simulink library "DelayLibrary"  (R2022b)
settings: Solver=VariableStepAuto  StartTime=0.0  StopTime=10.0  RelTol=1e-3
undefined symbols (not defined in the file or in its folder): Column, delay_chain, L, max_delay, num_input_chs
libraries: FeaturePath x4, AudioStats x4, RTC x3, TuneVar x3, $bdroot x2, ITC x2, dspsigops x1, TOP x1
(part 1 of 2)
settings Model: Creator=darshana.mistry  LastModifiedBy=kl13806
settings SolverCC: AlgebraicLoopSolver=TrustRegion
settings DebuggingCC: UnconnectedInputMsg=warning  UnconnectedOutputMsg=warning  UnconnectedLineMsg=warning  SFMachineParentedDataDiag=warning  ArithmeticOperatorsInVariantConditions=warning
settings ModelReferenceCC: EnableRefExpFcnMdlSchedulingChecks=on
settings SFSimCC: CustomCodeUndefinedFunction=UseInterfaceOnly
settings RTWCC: DLArmComputeVersion=19.05

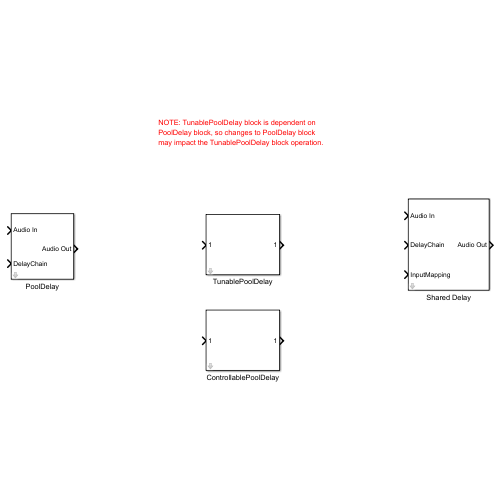
[thumbnail: Simulink's stored preview of the top-level diagram]
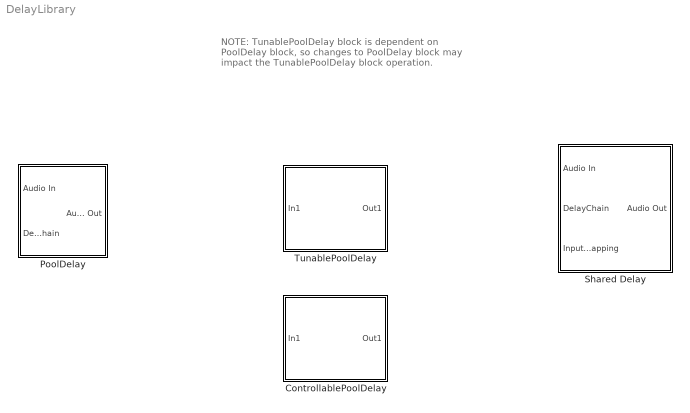
== system DelayLibrary ==
  note: NOTE: TunablePoolDelay block is dependent on
      | PoolDelay block, so changes to PoolDelay block
      | may impact the TunablePoolDelay block operation.
  ControllablePoolDelay : Subsystem  mask(Bose Tunable Pool Delay){delayType=In Samples, enableDelay=1, delaychain_var=delay_chain, maxTotalDelay=max_delay, frameSize=L, numChannels=num_input_chs, variantSelect=L2 Memory, PostOverlay=true, delayFrameLess=on, delayFrame=on, delayMultiFrame=on, FeatureName=ControllablePoolDelay, totalDelayBufferSize=0}
      mask prompts: delayType "Delay Type"; enableDelay "Enable Delay"; delaychain_var "Delay Chain for all channels (samples/ms)"; maxTotalDelay "Total Allotted Delay"; frameSize "Frame Size"; numChannels "Number Channels"; variantSelect "Implementation"; PostOverlay "Requires post-overlay action:"; delayFrameLess "delays <= frameSize"; delayFrame "frameSize < delays < (2 * frameSize)"; delayMultiFrame "delays >= (2 * frameSize)"; FeatureName "Delay name/purpose"; totalDelayBufferSize "Slow Delay Buffer Size"
      mask help:
      | 'Tunable Pool Delay' is based on 'Pool Delay' with addition of Tune and RTC parameter. Underlying block 'Pool Delay' is a multi-channel delay module with one single delay pool and adjustable delays per channel.
      | In this module, Delay chain is Tune parameter and Delay can be enabled or disabled via RTC message 'Enable_Delay'.
      mask TypeOptions delayType: In Samples | In Milliseconds
      mask TypeOptions maxTotalDelay: annDelaySubsystem/DelayEnableSubsystem/PoolDelay/maxTotalDelay | maxDelay/Value
      mask TypeOptions frameSize: annDelaySubsystem/DelayEnableSubsystem/PoolDelay/frameSize
      mask TypeOptions numChannels: annDelaySubsystem/DelayEnableSubsystem/PoolDelay/numChannels
      mask TypeOptions variantSelect: annDelaySubsystem/DelayEnableSubsystem/PoolDelay/variantSelect
      mask Callback variantSelect:
      | % Get the mask parameter value and container properties.
      | hMask = Simulink.Mask.get(gcb);
      | variant = get_param(gcb,'variantSelect');
      | container = hMask.getDialogControl('Container3');
      | 
      | % Check the value of 'variantSelect'
      | if strcmp(variant,"L2 Memory")
      |     % Set the visibility of delay panel
      |     container.Visible = 'on';
      |     MaskUtil.safe_setparam(gcbh, 'PostOverlay', 'true');
      | else
      |     % Set the visibility of delay panel
      |     container.Visible = 'off';
      |     MaskUtil.safe_setparam(gcbh, 'PostOverlay', 'false');
      | end
      mask TypeOptions PostOverlay: DelayTranslation/Delay_Samples/PostOverlay
      mask TypeOptions delayFrameLess: annDelaySubsystem/DelayEnableSubsystem/PoolDelay/delayFrameLess
      mask TypeOptions delayFrame: annDelaySubsystem/DelayEnableSubsystem/PoolDelay/delayFrame
      mask TypeOptions delayMultiFrame: annDelaySubsystem/DelayEnableSubsystem/PoolDelay/delayMultiFrame
      mask TypeOptions FeatureName: FeaturePath/FeatureName
      mask TypeOptions totalDelayBufferSize: annDelaySubsystem/DelayEnableSubsystem/PoolDelay/totalDelayBufferSize | annDelaySubsystem/DelayEnableSubsystem/PoolDelay/totalFastDelayBufferSize
      mask DialogControl Container3 Prompt: Delay Size Required
  PoolDelay : Subsystem  mask(Bose Pool Delay){variantSelect=L2 Memory, maxTotalDelay=512, delayFrameLess=on, delayFrame=on, delayMultiFrame=on, frameSize=32, numChannels=3, totalDelayBufferSize=0, totalFastDelayBufferSize=0}
      mask prompts: variantSelect "Implementation"; maxTotalDelay "Total Allotted Delay"; delayFrameLess "delays <= frameSize"; delayFrame "frameSize < delays < (2 * frameSize)"; delayMultiFrame "delays >= (2 * frameSize)"; frameSize "Frame Size"; numChannels "Number Channels"; totalDelayBufferSize "Slow Delay Buffer Size"; totalFastDelayBufferSize "Fast Delay Buffer Size"
      mask help:
      | Pool Delay is a multi-channel delay module with one single delay pool and adjustable delays per channel.  It provides support for delays greater than or equal to zero for one or more channels.  Total delay buffer size is the sum of all channel delays.  The Pool Delay model supports three different implementations, selectable from the model mask:
      |
      | - L1 Memory:  Optimized CRL (Code Replacement Library) code running on core with delay buffer in L1 Memory
      | - L2 Memory:  Optimized CRL code running on core and using DMA for memory copies with primary delay buffer in L2 Memory
      | - Generic:  Generic Matlab implementation running on core for targets without CRL support
      |
      | This model has two inputs and one output:
      |
      | - AudioIn [in]:  Audio input stream containing audio frame samples for one or more channels  [frameSize x numChannels]
      | - Delay [in]:  Delay in samples for each channel  [1 x numChannels]
      | - AudioOut [out]:  Audio output stream containing delayed audio frame samples for one or more channels  [frameSize x numChannels]
      |
      | NOTE: The Pool Delay codeWorkMemory buffer should always be mapped to L1 memory or core MIPS usage will increase.
      |
      | For more information, please see 'Help'.
      mask init:
      | % Create alias for delay buffer for each instance of model
      | PoolDelayMask(gcbh, variantSelect);
      | 
      | % There are three implementation types:
      | % Type    Value  Description
      | % L1 Memory  1      Optimized CRL code running on core with delay buffer
      | %                   in L1 Memory
      | % L2 Memory  2      Optimized CRL code running on core and using DMA for 
      | %                   memory copies with primary delay buffer in L2 Memory
      | % GENERIC    3      Generic Matlab implementation running on core for 
      | %                   other targets without CRL support
      | 
      | if variantSelect == 1
      |     % L1 Memory Core Implementation
      |     
      |     % Set delay buffer sizes. Only fast delay buffer (L1) is used for  
      |     % core implementation.
      |     totalFastDelayBufferSize = maxTotalDelay;
      |     totalDelayBufferSize =  2;      % Eliminates scaler CRL table entry
      |     
      |     % CRL code work memory size in bytes is equal to:
      |     %             sizeof(coreWorkMemory_t);
      |     % No variable data memory is used.  NOTE: This must be updated to 
      |     % match the CRL code if any changes are made to the coreWorkMemory_t 
      |     % structure.
      |     codeWorkMemorySize = (36/4);  % Size in words
      |     
      | elseif variantSelect == 2
      |     % L2 Memory DMA Implementation
      | 
      |     % Set delay buffer sizes. Total delay memory is split between
      |     % the delay buffer and fast delay buffer, with only 1 frame of
      |     % samples, or the delay (delay < frameSize) for each channel 
      |     % stored in the fast delay buffer. Get the delay buffer sizes and
      |     % DMA TCB memory required for the worst case Room Mode Down Load
      |     % given the specified delay categories and maxTotalDelay.
      |     delayConfig = [delayFrameLess, delayFrame, delayMultiFrame];
      |     [totalFastDelayBufferSize, totalDelayBufferSize, ...
      |      maxTcbMemSize, maxChanMapSize] = ...
      |             PoolDelayDmaMemorySizes(delayConfig, maxTotalDelay, ...
      |                                     numChannels, frameSize);
      |     
      |     % Make sure circular delay buffer size is at least as large as the
      |     % frame size. Note this is required to ensure the SHARC built-in
      |     % circindex() function works correctly in the CRL code.
      |     totalDelayBufferSize = max(frameSize, totalDelayBufferSize);
      |     
      |     % CRL code work memory size in bytes is equal to:
      |     %             sizeof(dmaWorkMemory_t) + variableDataSize;
      |     % with variable data size dependent on number channels and number
      |     % DMA TCB blocks.  NOTE: This must be updated to match the CRL code
      |     % if any changes are made to the dmaWorkMemory_t structure.
      |     codeWorkMemorySize = (156/4) + maxTcbMemSize + maxChanMapSize; % Size in words
      |     
      | else
      |     % Generic Implementation
      |     
      |     % Set delay buffer sizes. Only fast delay buffer (L1) is used for
      |     % generic implementation.
      |     totalFastDelayBufferSize = maxTotalDelay;
      |     totalDelayBufferSize =  1;    
      |     
      |     % This is not used if there is no CRL
      |     codeWorkMemorySize = 1;
      | end
      mask Help:
      | Help on Mask Parameters:
      | 
      | All variants of the model contain the following mask parameters:
      | 
      | - Implementation:  Selects the desired model implementation to use (L1 Memory, L2 Memory, or Generic)
      | - Total Allotted Delay:  The provides delay buffer sizing for the maximum Room Model Down Load (RMDL) or non-RMDL delay configuration required.  It is the sum of all channels delays in samples for the largest RMDL delay case.  (scalar)
      | - Frame Size:  Specifies the audio frame size in samples (scalar)
      | - Number Channels:  Specifies the number of channel and applies to the audio input, output, and delay channels (scalar)
      | 
      | The 'L2 Memory' implementation contains the following additional mask parameter:
      | 
      | - Delay Sizes Required: The appropriate check boxes must be checked to specify delay categories required.  Delay categories include the following: (delays <= frameSize), (frameSize < delays < (2 * frameSize)), and (delays >= (2 * frameSize).  The correct selection of these delay categories is required to ensure the delay buffers and other model data is sized correctly.
      | 
      | Note that since the 'L2 Memory' implementations takes advantage of DMA memory copies performed by the hardware DMA engine, the implementation differs from the other model implementations and in order to minimize the memory usage required to support all channel delay configurations, the channel delay categories required must be known.  The specific delay cases required for RMDL and non-RMDL model instances determine overall memory required for delay buffers and DMA descriptor memory.
      | 
      | Mask Usage Example:
      | 
      | 3 input and output channels, with channel delays of 16, 48, 80 samples for a case that does not require RMDL, and a frame size of 32 samples.
      | 
      | For example, to use the  L1 Memory implementation, set the mask parameters as follows:
      | 
      | Implementation = 'L1 Memory'
      | Total RMDL Allotted Delay = 148        (16 + 48 + 80)
      | Frame Size = 32
      | Number Channels = 3
      | 
      | For the same example with the L2 Memory implementation, set all the above parameters as stated, except with:
      | 
      | Implementation = 'L2 Memory'
      | Delay Sizes Required should have all delay categories checked, as the delays of 16, 48, 80 include all categories.  These parameters and the Total Allotted Delay are used size memory to support the delay configuration.  If for example, all delays required were less than equal to a frame only that delay category should be checked.
      | 
      | Note that 'Delay Sizes Required' is specific to the L2 Memory implementation and does not apply to the other implementations.
      | 
      | The 'Generic' implementation would require the identical mask parameter initialization as the L1 memory implementation, except with:
      | 
      | Implementation = 'Generic'
      mask TypeOptions variantSelect: L1 Memory | L2 Memory | Generic
      mask Callback variantSelect:
      | % Get the mask parameter value and container properties.
      | hMask = Simulink.Mask.get(gcb);
      | variant = get_param(gcb,'variantSelect');
      | container = hMask.getDialogControl('DelayPanel');
      | 
      | % Check the value of 'variantSelect'
      | if strcmp(variant,"L2 Memory")
      |     % Set the visibility of delay panel
      |     container.Visible = 'on';
      | else
      |     % Set the visibility of delay panel
      |     container.Visible = 'off';
      | end
      mask DialogControl DelayPanel Prompt: Delay Sizes Required
  Shared Delay : Subsystem  mask(Bose Shared Delay){maxTotalDelay=512, frameSize=32, numInputs=2, numOutputs=3, totalDelayBufferSize=0, fastDmaBufferSize=0}
      mask prompts: maxTotalDelay "Total Allotted Delay"; frameSize "Frame Size"; numInputs "Number Inputs"; numOutputs "Number Outputs"; totalDelayBufferSize "Slow Delay Buffer Size"; fastDmaBufferSize "Fast DMA Buffer Size"
      mask help:
      | Shared Delay is a multi-input channel delay module with one or more adjustable output delay taps per input channel, based on how input channels are mapped to outputs.  It provides support for delays greater than or equal to zero.  The Shared Delay model supports only one implementation.  It is a DMA based write before delay buffer read implementation, with total delay buffer size of the sum of the maximum output channel tap delay for each input channel, plus one frame size per input channel.
      |
      | This model has two inputs and one output:
      |
      | - AudioIn [in]:  Audio input stream containing audio frame samples for one or more input channels  [frameSize x numInputs]
      | - DelayChain [in]:  Delay in samples for all input channel's output tap channels  [1 x numOutputs]
      | - InputMapping [in]:  Zero based mapping of input channels to output tap channels  [1 x numOutputs]
      | - AudioOut [out]:  Audio output stream containing delayed audio frame samples for one or more output channels  [frameSize x numOutputs]
      |
      | The delay buffer can be mapped to L3, L2 or L1 memory with proper definition of the code generated pragma section memory mappings.
      |
      | NOTE: The Shared Delay codeWorkMemory buffer should always be mapped to L1 memory or core MIPS usage will increase.
      |
      | For more information, please see 'Help'.
      mask init:
      | % Create alias for delay buffer for each instance of model
      | SharedDelayMask(gcbh);
      | 
      | % Set delay buffer size and fast DMA output buffer size. These
      | % are worst case Room Mode Down Load sizes given maxTotalDelay.
      | totalDelayBufferSize = maxTotalDelay + (numInputs * frameSize);
      | fastDmaBufferSize = numOutputs * frameSize;
      | 
      | % CRL code work memory size in bytes is equal to:
      | %             sizeof(dmaWorkMemory_t) + variableDataSize;
      | % with variable data size dependent on number channels and number
      | % DMA TCB blocks.  NOTE: This must be updated to match the CRL code
      | % if any changes are made to the dmaWorkMemory_t structure.
      | codeWorkMemorySize = (160/4) + (numInputs * (14 + 5)) + ...
      |                      (2 * numOutputs);    % Size in words
      mask Help:
      | Help on Mask Parameters:
      | 
      | The Shared Delay model contains the following mask parameters:
      | 
      | - Total Allotted Delay:  Specifies delay buffer sizing for the maximum Room Model Down Load (RMDL) or non-RMDL delay configuration required.  It is the sum of the maximum output channel tap delay for each input channel in samples that supports the largest RMDL delay case.  (scalar)
      | - Frame Size:  Specifies the audio frame size in samples (scalar)
      | - Number Input Channels:  Specifies the number of input channels and applies to the audio inputs (scalar)
      | - Number Output Channels:  Specifies the number of output channels and applies to the audio outputs, delays and input mapping (scalar)
      | 
      | Mask Usage Example:
      | 
      | 2 input channels, with output channel tap delays of 16, 48, 80 samples for input 1 and output channel tap delays of 37, 62 samples for input channel 2.    Assumption is this case does not require RMDL and the frame size is 32 samples.
      | 
      | For this example, set the mask parameters and inputs as follows:
      | 
      | Total Allotted Delay = 142        max( [16 48 80] ) + max( [37  62] ) = 80 + 62
      | Frame Size = 32
      | Number Inputs = 2
      | Number Outputs = 5                (3 + 2)
      | 
      | DelayChain = [16 48 80 37 62]
      | InputMapping = [0 0 0 1 1]
  TunablePoolDelay : Subsystem  mask(Bose Tunable Pool Delay){delayType=In Samples, enableDelay=1, delaychain_var=delay_chain, maxTotalDelay=max_delay, frameSize=L, numChannels=num_input_chs, variantSelect=L2 Memory, PostOverlay=true, delayFrameLess=on, delayFrame=on, delayMultiFrame=on, FeatureName=TunablePoolDelay, totalDelayBufferSize=0}
      mask prompts: delayType "Delay Type"; enableDelay "Enable Delay"; delaychain_var "Delay Chain for all channels (samples/ms)"; maxTotalDelay "Total Allotted Delay"; frameSize "Frame Size"; numChannels "Number Channels"; variantSelect "Implementation"; PostOverlay "Requires post-overlay action:"; delayFrameLess "delays <= frameSize"; delayFrame "frameSize < delays < (2 * frameSize)"; delayMultiFrame "delays >= (2 * frameSize)"; FeatureName "Delay name/purpose"; totalDelayBufferSize "Slow Delay Buffer Size"
      mask help:
      | 'Tunable Pool Delay' is based on 'Pool Delay' with addition of Tune and RTC parameter. Underlying block 'Pool Delay' is a multi-channel delay module with one single delay pool and adjustable delays per channel.
      | In this module, Delay chain is Tune parameter and Delay can be enabled or disabled via RTC message 'Enable_Delay'.
      mask TypeOptions delayType: In Samples | In Milliseconds
      mask TypeOptions maxTotalDelay: annDelaySubsystem/DelayEnableSubsystem/PoolDelay/maxTotalDelay | maxDelay/Value
      mask TypeOptions frameSize: annDelaySubsystem/DelayEnableSubsystem/PoolDelay/frameSize
      mask TypeOptions numChannels: annDelaySubsystem/DelayEnableSubsystem/PoolDelay/numChannels
      mask TypeOptions variantSelect: annDelaySubsystem/DelayEnableSubsystem/PoolDelay/variantSelect
      mask Callback variantSelect:
      | % Get the mask parameter value and container properties.
      | hMask = Simulink.Mask.get(gcb);
      | variant = get_param(gcb,'variantSelect');
      | container = hMask.getDialogControl('Container3');
      | 
      | % Check the value of 'variantSelect'
      | if strcmp(variant,"L2 Memory")
      |     % Set the visibility of delay panel
      |     container.Visible = 'on';
      |     MaskUtil.safe_setparam(gcbh, 'PostOverlay', 'true');
      | else
      |     % Set the visibility of delay panel
      |     container.Visible = 'off';
      |     MaskUtil.safe_setparam(gcbh, 'PostOverlay', 'false');
      | end
      mask TypeOptions PostOverlay: DelayTranslation/Delay_Samples/PostOverlay
      mask TypeOptions delayFrameLess: annDelaySubsystem/DelayEnableSubsystem/PoolDelay/delayFrameLess
      mask TypeOptions delayFrame: annDelaySubsystem/DelayEnableSubsystem/PoolDelay/delayFrame
      mask TypeOptions delayMultiFrame: annDelaySubsystem/DelayEnableSubsystem/PoolDelay/delayMultiFrame
      mask TypeOptions FeatureName: FeaturePath/FeatureName
      mask TypeOptions totalDelayBufferSize: annDelaySubsystem/DelayEnableSubsystem/PoolDelay/totalDelayBufferSize | annDelaySubsystem/DelayEnableSubsystem/PoolDelay/totalFastDelayBufferSize
      mask DialogControl Container3 Prompt: Delay Size Required

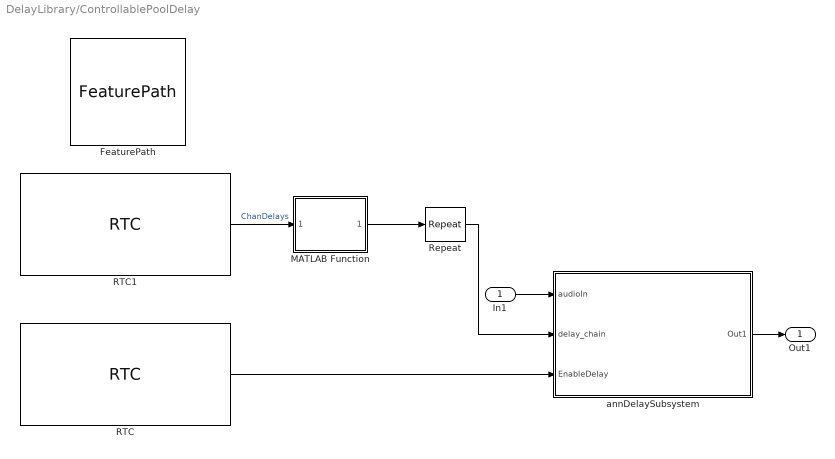
== system DelayLibrary/ControllablePoolDelay ==
  In1 : Inport
  FeaturePath : FeaturePath/FeaturePath  FeatureName=ControllablePoolDelay  IsGroup=off  GroupNumber=-1  IsModule=off  TriggerInit=[-120 -76 -5 31]
      settings: SourceProductName=Bose Talaria
  MATLAB Function : MATLAB Function  TreatAsAtomicUnit=on
  RTC : RTC/RTC  REQ_Priority=RTC_Mask.NormalPriority  RequestAtInit=off  EnableRequest=off  REQElemName1=Enable_annDelay  REQElemType1=uint32  REQElemWidth1=1  REQElemInitial1=enableDelay  REQElemType2=uint32  REQElemWidth2=1  REQElemInitial2=[]  REQElemType3=uint32  REQElemWidth3=1  REQElemInitial3=[]  REQElemType4=uint32  REQElemWidth4=1  REQElemInitial4=[]  REQElemType5=uint32  REQElemWidth5=1  REQElemInitial5=[]  REQElemType6=uint32  REQElemWidth6=1  REQElemInitial6=[]  REQElemType7=uint32  REQElemWidth7=1  REQElemInitial7=[]  REQElemType8=uint32  REQElemWidth8=1  REQElemInitial8=[]  REQElemType9=uint32  REQElemWidth9=1  REQElemInitial9=[]  REQElemType10=uint32  REQElemWidth10=1  REQElemInitial10=[]  EnableResponse=on  EnableRSP_StatusIn=off  RSPElemType1=uint32  RSPElemWidth1=1  RSPElemType2=uint32  RSPElemWidth2=1  RSPElemType3=uint32  RSPElemWidth3=1  RSPElemType4=uint32  RSPElemWidth4=1  RSPElemType5=uint32  RSPElemWidth5=1  RSPElemType6=uint32  RSPElemWidth6=1  RSPElemType7=uint32  RSPElemWidth7=1  RSPElemType8=uint32  RSPElemWidth8=1  RSPElemType9=uint32  RSPElemWidth9=1  RSPElemType10=uint32  RSPElemWidth10=1  EnableNotification=off  EnableNTF_PrepTrig=off  NTFElemType1=uint32  NTFElemWidth1=1  NTFElemType2=uint32  NTFElemWidth2=1  NTFElemType3=uint32  NTFElemWidth3=1  NTFElemType4=uint32  NTFElemWidth4=1  NTFElemType5=uint32  NTFElemWidth5=1  NTFElemType6=uint32  NTFElemWidth6=1  NTFElemType7=uint32  NTFElemWidth7=1  NTFElemType8=uint32  NTFElemWidth8=1  NTFElemType9=uint32  NTFElemWidth9=1  NTFElemType10=uint32  NTFElemWidth10=1  MaskMessageName=Enable_Delay
      settings: SourceProductName=Bose Talaria
  RTC1 : RTC/RTC  REQ_Priority=RTC_Mask.NormalPriority  RequestAtInit=off  EnableRequest=off  REQElemName1=Delay_value  REQElemType1=uint32  REQElemWidth1=1  REQElemInitial1=delaychain_var  REQElemType2=uint32  REQElemWidth2=1  REQElemInitial2=[]  REQElemType3=uint32  REQElemWidth3=1  REQElemInitial3=[]  REQElemType4=uint32  REQElemWidth4=1  REQElemInitial4=[]  REQElemType5=uint32  REQElemWidth5=1  REQElemInitial5=[]  REQElemType6=uint32  REQElemWidth6=1  REQElemInitial6=[]  REQElemType7=uint32  REQElemWidth7=1  REQElemInitial7=[]  REQElemType8=uint32  REQElemWidth8=1  REQElemInitial8=[]  REQElemType9=uint32  REQElemWidth9=1  REQElemInitial9=[]  REQElemType10=uint32  REQElemWidth10=1  REQElemInitial10=[]  EnableResponse=on  EnableRSP_StatusIn=off  RSPElemType1=uint32  RSPElemWidth1=1  RSPElemType2=uint32  RSPElemWidth2=1  RSPElemType3=uint32  RSPElemWidth3=1  RSPElemType4=uint32  RSPElemWidth4=1  RSPElemType5=uint32  RSPElemWidth5=1  RSPElemType6=uint32  RSPElemWidth6=1  RSPElemType7=uint32  RSPElemWidth7=1  RSPElemType8=uint32  RSPElemWidth8=1  RSPElemType9=uint32  RSPElemWidth9=1  RSPElemType10=uint32  RSPElemWidth10=1  EnableNotification=off  EnableNTF_PrepTrig=off  NTFElemType1=uint32  NTFElemWidth1=1  NTFElemType2=uint32  NTFElemWidth2=1  NTFElemType3=uint32  NTFElemWidth3=1  NTFElemType4=uint32  NTFElemWidth4=1  NTFElemType5=uint32  NTFElemWidth5=1  NTFElemType6=uint32  NTFElemWidth6=1  NTFElemType7=uint32  NTFElemWidth7=1  NTFElemType8=uint32  NTFElemWidth8=1  NTFElemType9=uint32  NTFElemWidth9=1  NTFElemType10=uint32  NTFElemWidth10=1  MaskMessageName=Delay_value
      settings: SourceProductName=Bose Talaria
  Repeat : dspsigops/Repeat  N=numChannels  InputProcessing=Columns as channels (frame based)  RateOptions=Enforce single-rate processing  ic=0  mode=Unused parameter value
  annDelaySubsystem : Subsystem
  Out1 : Outport  VectorParamsAs1DForOutWhenUnconnected=off
  wires:
  In1/1 -> annDelaySubsystem/1(audioIn)
  annDelaySubsystem/1(Out1) -> Out1/1
  RTC1/1 -> MATLAB Function/1(Amount)  "ChanDelays"
  Repeat/1 -> annDelaySubsystem/2(delay_chain)
  RTC/1 -> annDelaySubsystem/3(EnableDelay)
  MATLAB Function/1(Samples) -> Repeat/1

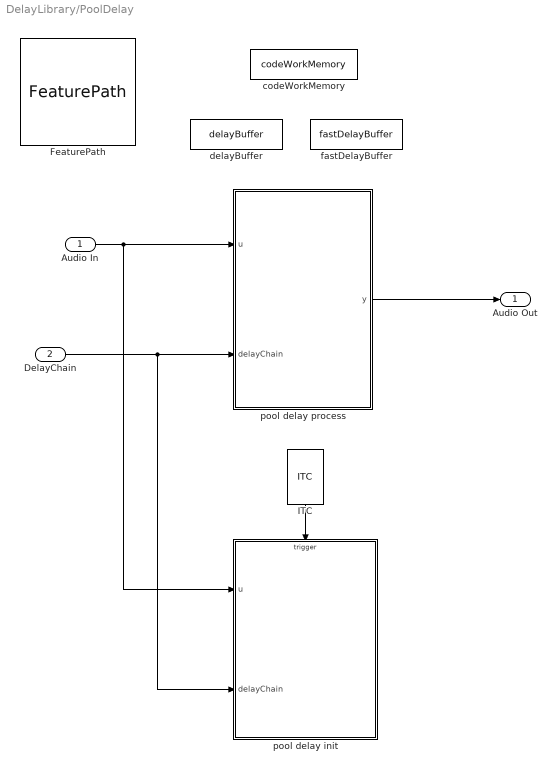
== system DelayLibrary/PoolDelay ==
  Audio In : Inport
  DelayChain : Inport  Port=2  OutDataTypeStr=uint32  PortDimensions=[1, numChannels]
  FeaturePath : FeaturePath/FeaturePath  FeatureName=PoolDelay  IsGroup=off  GroupNumber=-1  IsModule=off  TriggerInit=[205 -116 320 -9]
      settings: SourceProductName=Bose Talaria
  ITC : ITC/ITC
      settings: SourceProductName=Bose Talaria
  codeWorkMemory : DataStoreMemory  DataStoreName=codeWorkMemory  WriteAfterWriteMsg=warning  InitialValue=zeros(1,codeWorkMemorySize)  EmbeddedSignalClassName=Blocklib.Signal  ShowAdditionalParam=off  OutDataTypeStr=uint32
  delayBuffer : DataStoreMemory  DataStoreName=delayBuffer  ReadBeforeWriteMsg=warning  WriteAfterWriteMsg=warning  WriteAfterReadMsg=warning  InitialValue=zeros(totalDelayBufferSize,1)  EmbeddedSignalClassName=Blocklib.Signal  ShowAdditionalParam=off  OutDataTypeStr=single
  fastDelayBuffer : DataStoreMemory  DataStoreName=fastDelayBuffer  ReadBeforeWriteMsg=warning  WriteAfterWriteMsg=warning  WriteAfterReadMsg=warning  InitialValue=zeros(totalFastDelayBufferSize,1)  EmbeddedSignalClassName=Blocklib.Signal  ShowAdditionalParam=off  OutDataTypeStr=single
  pool delay init : MATLAB Function  TreatAsAtomicUnit=on  RTWFcnName=foo
  pool delay process : MATLAB Function  TreatAsAtomicUnit=on
  Audio Out : Outport  VectorParamsAs1DForOutWhenUnconnected=off
  wires:
  ITC/1 -> pool delay init/Trigger
  pool delay process/1(y) -> Audio Out/1
  Audio In/1 -> pool delay process/1(u), pool delay init/1(u)
  DelayChain/1 -> pool delay init/2(delayChain), pool delay process/2(delayChain)

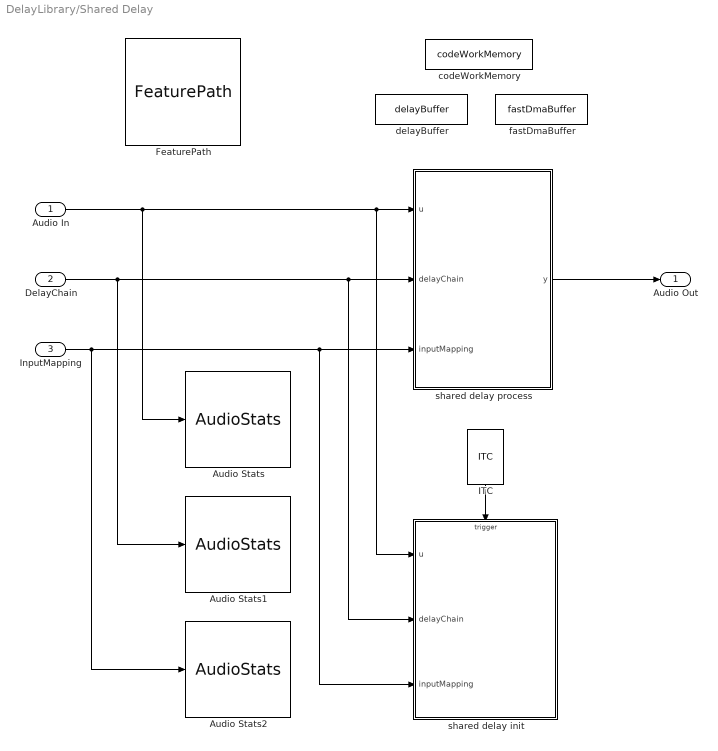
== system DelayLibrary/Shared Delay ==
  Audio In : Inport
  DelayChain : Inport  Port=2  OutDataTypeStr=int32  PortDimensions=[1, numOutputs]
  InputMapping : Inport  Port=3  OutDataTypeStr=int32  PortDimensions=[1 numOutputs]
  Audio Stats : AudioStats/AudioStats  DoSampleRate=off  TypeSampleRate=Inherit: auto  DoCallRate=off  TypeCallRate=Inherit: auto  DoFrameSize=off  TypeFrameSize=Inherit: auto  DoChannelCount=off  TypeChannelCount=Inherit: auto  DoTaskRateFactor=off  TypeTaskRateFactor=Inherit: auto  MacroNameRoot=AUDIO  MacroNameRootEval='AUDIO'  IsMacroNameEval=off  MacroSampleRate=off  MacroCallRate=off  MacroFrameSize=off  MacroChannelCount=off  MacroTaskRateFactor=off  MacroTaskId=off  ValidateSampleRate=off  ValueSampleRate=[]  ValidateCallRate=off  ValueCallRate=[]  ValidateFrameSize=on  ValueFrameSize=frameSize  ValidateChannelCount=on  ValueChannelCount=numInputs  ValidateTaskRateFactor=off  ValueTaskRateFactor=[]
      settings: SourceProductName=Bose Talaria
  Audio Stats1 : AudioStats/AudioStats  DoSampleRate=off  TypeSampleRate=Inherit: auto  DoCallRate=off  TypeCallRate=Inherit: auto  DoFrameSize=off  TypeFrameSize=Inherit: auto  DoChannelCount=off  TypeChannelCount=Inherit: auto  DoTaskRateFactor=off  TypeTaskRateFactor=Inherit: auto  MacroNameRoot=AUDIO  MacroNameRootEval='AUDIO'  IsMacroNameEval=off  MacroSampleRate=off  MacroCallRate=off  MacroFrameSize=off  MacroChannelCount=off  MacroTaskRateFactor=off  MacroTaskId=off  ValidateSampleRate=off  ValueSampleRate=[]  ValidateCallRate=off  ValueCallRate=[]  ValidateFrameSize=off  ValueFrameSize=[]  ValidateChannelCount=on  ValueChannelCount=numOutputs  ValidateTaskRateFactor=off  ValueTaskRateFactor=[]
      settings: SourceProductName=Bose Talaria
  Audio Stats2 : AudioStats/AudioStats  DoSampleRate=off  TypeSampleRate=Inherit: auto  DoCallRate=off  TypeCallRate=Inherit: auto  DoFrameSize=off  TypeFrameSize=Inherit: auto  DoChannelCount=off  TypeChannelCount=Inherit: auto  DoTaskRateFactor=off  TypeTaskRateFactor=Inherit: auto  MacroNameRoot=AUDIO  MacroNameRootEval='AUDIO'  IsMacroNameEval=off  MacroSampleRate=off  MacroCallRate=off  MacroFrameSize=off  MacroChannelCount=off  MacroTaskRateFactor=off  MacroTaskId=off  ValidateSampleRate=off  ValueSampleRate=[]  ValidateCallRate=off  ValueCallRate=[]  ValidateFrameSize=off  ValueFrameSize=[]  ValidateChannelCount=on  ValueChannelCount=numOutputs  ValidateTaskRateFactor=off  ValueTaskRateFactor=[]
      settings: SourceProductName=Bose Talaria
  FeaturePath : FeaturePath/FeaturePath  FeatureName=SharedDelay  IsGroup=off  GroupNumber=-1  IsModule=off  TriggerInit=[310 -96 425 11]
      settings: SourceProductName=Bose Talaria
  ITC : ITC/ITC
      settings: SourceProductName=Bose Talaria
  codeWorkMemory : DataStoreMemory  DataStoreName=codeWorkMemory  WriteAfterWriteMsg=warning  InitialValue=zeros(1,codeWorkMemorySize)  EmbeddedSignalClassName=Blocklib.Signal  ShowAdditionalParam=off  OutDataTypeStr=uint32
  delayBuffer : DataStoreMemory  DataStoreName=delayBuffer  ReadBeforeWriteMsg=warning  WriteAfterWriteMsg=warning  WriteAfterReadMsg=warning  InitialValue=zeros(totalDelayBufferSize,1)  EmbeddedSignalClassName=Blocklib.Signal  ShowAdditionalParam=off  OutDataTypeStr=single
  fastDmaBuffer : DataStoreMemory  DataStoreName=fastDmaBuffer  ReadBeforeWriteMsg=warning  WriteAfterWriteMsg=warning  WriteAfterReadMsg=warning  InitialValue=zeros(fastDmaBufferSize,1)  EmbeddedSignalClassName=Blocklib.Signal  ShowAdditionalParam=off  OutDataTypeStr=single
  shared delay init : MATLAB Function  TreatAsAtomicUnit=on  RTWFcnName=foo
  shared delay process : MATLAB Function  TreatAsAtomicUnit=on
  Audio Out : Outport  VectorParamsAs1DForOutWhenUnconnected=off
  wires:
  Audio In/1 -> shared delay process/1(u), shared delay init/1(u), Audio Stats/1
  InputMapping/1 -> shared delay process/3(inputMapping), shared delay init/3(inputMapping), Audio Stats2/1
  ITC/1 -> shared delay init/Trigger
  shared delay process/1(y) -> Audio Out/1
  DelayChain/1 -> shared delay process/2(delayChain), shared delay init/2(delayChain), Audio Stats1/1

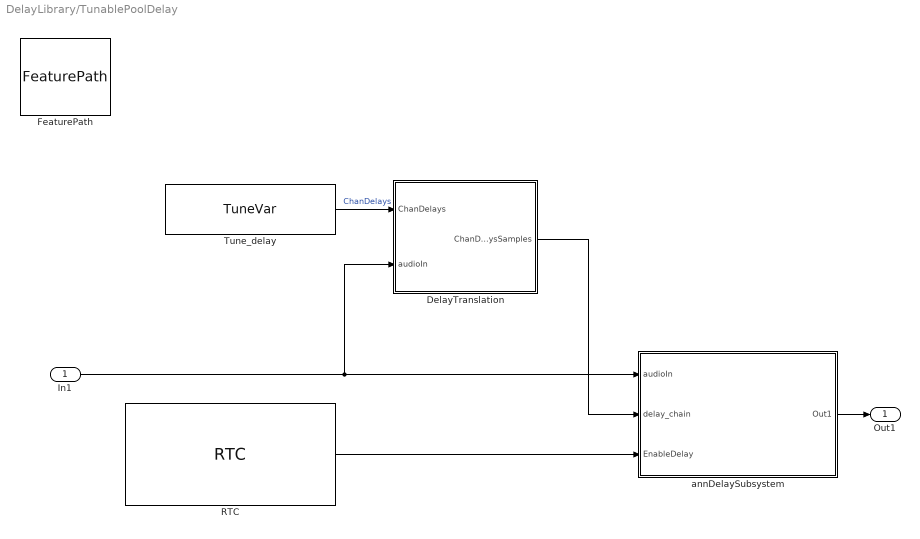
== system DelayLibrary/TunablePoolDelay ==
  In1 : Inport
  DelayTranslation : Subsystem
  FeaturePath : FeaturePath/FeaturePath  FeatureName=TunablePoolDelay  IsGroup=off  GroupNumber=-1  IsModule=off  TriggerInit=[-255 -156 -165 -79]
      settings: SourceProductName=Bose Talaria
  RTC : RTC/RTC  REQ_Priority=RTC_Mask.NormalPriority  RequestAtInit=off  EnableRequest=off  REQElemName1=Enable_annDelay  REQElemType1=uint32  REQElemWidth1=1  REQElemInitial1=enableDelay  REQElemType2=uint32  REQElemWidth2=1  REQElemInitial2=[]  REQElemType3=uint32  REQElemWidth3=1  REQElemInitial3=[]  REQElemType4=uint32  REQElemWidth4=1  REQElemInitial4=[]  REQElemType5=uint32  REQElemWidth5=1  REQElemInitial5=[]  REQElemType6=uint32  REQElemWidth6=1  REQElemInitial6=[]  REQElemType7=uint32  REQElemWidth7=1  REQElemInitial7=[]  REQElemType8=uint32  REQElemWidth8=1  REQElemInitial8=[]  REQElemType9=uint32  REQElemWidth9=1  REQElemInitial9=[]  REQElemType10=uint32  REQElemWidth10=1  REQElemInitial10=[]  EnableResponse=on  EnableRSP_StatusIn=off  RSPElemType1=uint32  RSPElemWidth1=1  RSPElemType2=uint32  RSPElemWidth2=1  RSPElemType3=uint32  RSPElemWidth3=1  RSPElemType4=uint32  RSPElemWidth4=1  RSPElemType5=uint32  RSPElemWidth5=1  RSPElemType6=uint32  RSPElemWidth6=1  RSPElemType7=uint32  RSPElemWidth7=1  RSPElemType8=uint32  RSPElemWidth8=1  RSPElemType9=uint32  RSPElemWidth9=1  RSPElemType10=uint32  RSPElemWidth10=1  EnableNotification=off  EnableNTF_PrepTrig=off  NTFElemType1=uint32  NTFElemWidth1=1  NTFElemType2=uint32  NTFElemWidth2=1  NTFElemType3=uint32  NTFElemWidth3=1  NTFElemType4=uint32  NTFElemWidth4=1  NTFElemType5=uint32  NTFElemWidth5=1  NTFElemType6=uint32  NTFElemWidth6=1  NTFElemType7=uint32  NTFElemWidth7=1  NTFElemType8=uint32  NTFElemWidth8=1  NTFElemType9=uint32  NTFElemWidth9=1  NTFElemType10=uint32  NTFElemWidth10=1  MaskMessageName=Enable_Delay
      settings: SourceProductName=Bose Talaria
  Tune_delay : TuneVar/TuneVar  TuneName=ChanDelays  SpecifyMaxSize=off  VariableDim=2 (Column)  MaxSize=[1 1]  TunabilityNumber=1  MinValue=[]  MaxValue=[]  TriggerInit=[-110 -10 60 40]  MaskValue=delaychain_var
      settings: SourceProductName=Bose Talaria
  annDelaySubsystem : Subsystem
  Out1 : Outport  VectorParamsAs1DForOutWhenUnconnected=off
  wires:
  RTC/1 -> annDelaySubsystem/3(EnableDelay)
  DelayTranslation/1(ChanDelaysSamples) -> annDelaySubsystem/2(delay_chain)
  Tune_delay/1 -> DelayTranslation/1(ChanDelays)  "ChanDelays"
  annDelaySubsystem/1(Out1) -> Out1/1
  In1/1 -> annDelaySubsystem/1(audioIn), DelayTranslation/2(audioIn)

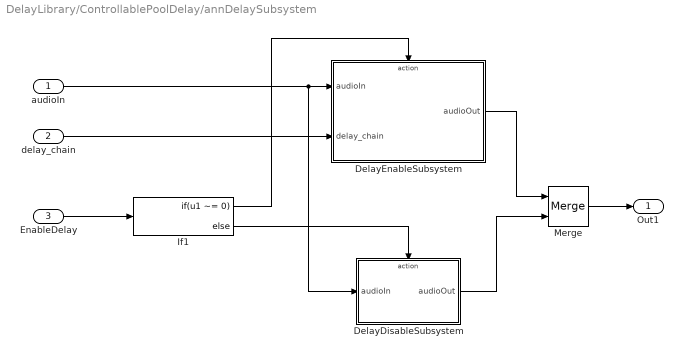
== system DelayLibrary/ControllablePoolDelay/annDelaySubsystem ==
  audioIn : Inport
  delay_chain : Inport  Port=2
  EnableDelay : Inport  Port=3
  DelayDisableSubsystem : Subsystem  TreatAsAtomicUnit=on
  DelayEnableSubsystem : Subsystem  TreatAsAtomicUnit=on
  If1 : If  IfExpression=u1 ~= 0
  Merge : Merge
  Out1 : Outport  VectorParamsAs1DForOutWhenUnconnected=off
  wires:
  EnableDelay/1 -> If1/1
  If1/1 -> DelayEnableSubsystem/Action
  audioIn/1 -> DelayDisableSubsystem/1(audioIn), DelayEnableSubsystem/1(audioIn)
  delay_chain/1 -> DelayEnableSubsystem/2(delay_chain)
  DelayEnableSubsystem/1(audioOut) -> Merge/1
  If1/2 -> DelayDisableSubsystem/Action
  Merge/1 -> Out1/1
  DelayDisableSubsystem/1(audioOut) -> Merge/2

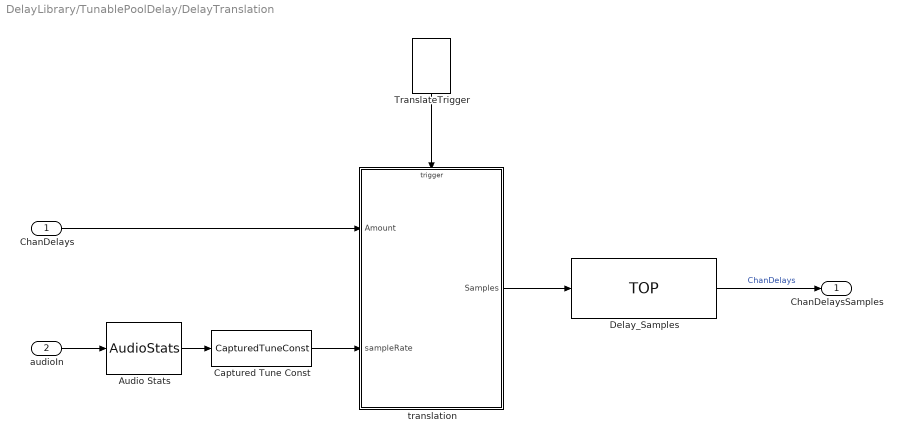
== system DelayLibrary/TunablePoolDelay/DelayTranslation ==
  ChanDelays : Inport
  audioIn : Inport  Port=2
  Audio Stats : AudioStats/AudioStats  DoSampleRate=on  TypeSampleRate=Inherit: auto  DoCallRate=off  TypeCallRate=Inherit: auto  DoFrameSize=off  TypeFrameSize=Inherit: auto  DoChannelCount=off  TypeChannelCount=Inherit: auto  DoTaskRateFactor=off  TypeTaskRateFactor=Inherit: auto  MacroNameRoot=AUDIO  MacroNameRootEval='AUDIO'  IsMacroNameEval=off  MacroSampleRate=off  MacroCallRate=off  MacroFrameSize=off  MacroChannelCount=off  MacroTaskRateFactor=off  MacroTaskId=off  ValidateSampleRate=off  ValueSampleRate=[]  ValidateCallRate=off  ValueCallRate=[]  ValidateFrameSize=off  ValueFrameSize=[]  ValidateChannelCount=off  ValueChannelCount=[]  ValidateTaskRateFactor=off  ValueTaskRateFactor=[]
      settings: SourceProductName=Bose Talaria
  Captured Tune Const : TuneVar/CapturedTuneConst  TriggerInit=[205 312 305 348]  Role=Automatic
      settings: SourceProductName=Bose Talaria
  Delay_Samples : TOP/TOP  TriggerInit=[565 240 710 300]  TopName=ChanDelays  DataType=uint32  BankNumber=0  PreOverlay=false  PostOverlay=PostOverlay  Role=Automatic
      settings: SourceProductName=Bose Talaria
  TranslateTrigger : TuneVar/TranslateTrigger  TriggerInit=[406 20 444 75]
      settings: SourceProductName=Bose Talaria
  translation : MATLAB Function  TreatAsAtomicUnit=on
  ChanDelaysSamples : Outport  VectorParamsAs1DForOutWhenUnconnected=off
  wires:
  audioIn/1 -> Audio Stats/1
  Delay_Samples/1 -> ChanDelaysSamples/1  "ChanDelays"
  TranslateTrigger/1 -> translation/Trigger
  Captured Tune Const/1 -> translation/2(sampleRate)
  ChanDelays/1 -> translation/1(Amount)
  translation/1(Samples) -> Delay_Samples/1
  Audio Stats/1 -> Captured Tune Const/1

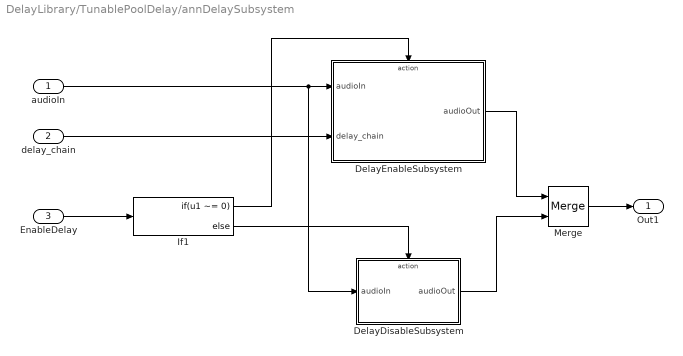
== system DelayLibrary/TunablePoolDelay/annDelaySubsystem ==
  audioIn : Inport
  delay_chain : Inport  Port=2
  EnableDelay : Inport  Port=3
  DelayDisableSubsystem : Subsystem  TreatAsAtomicUnit=on
  DelayEnableSubsystem : Subsystem  TreatAsAtomicUnit=on
  If1 : If  IfExpression=u1 ~= 0
  Merge : Merge
  Out1 : Outport  VectorParamsAs1DForOutWhenUnconnected=off
  wires:
  DelayDisableSubsystem/1(audioOut) -> Merge/2
  Merge/1 -> Out1/1
  If1/2 -> DelayDisableSubsystem/Action
  DelayEnableSubsystem/1(audioOut) -> Merge/1
  delay_chain/1 -> DelayEnableSubsystem/2(delay_chain)
  audioIn/1 -> DelayEnableSubsystem/1(audioIn), DelayDisableSubsystem/1(audioIn)
  If1/1 -> DelayEnableSubsystem/Action
  EnableDelay/1 -> If1/1

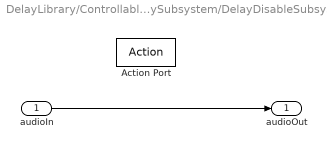
== system DelayLibrary/ControllablePoolDelay/annDelaySubsystem/DelayDisableSubsystem ==
  audioIn : Inport
  Action Port : ActionPort
  audioOut : Outport  VectorParamsAs1DForOutWhenUnconnected=off
  wires:
  audioIn/1 -> audioOut/1

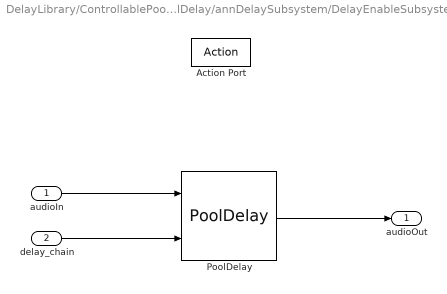
== system DelayLibrary/ControllablePoolDelay/annDelaySubsystem/DelayEnableSubsystem ==
  audioIn : Inport
  delay_chain : Inport  Port=2
  Action Port : ActionPort
  PoolDelay : $bdroot/PoolDelay  variantSelect=L2 Memory  maxTotalDelay=maxTotalDelay  delayFrameLess=on  delayFrame=on  delayMultiFrame=on  frameSize=frameSize  numChannels=numChannels  totalDelayBufferSize=totalDelayBufferSize  totalFastDelayBufferSize=totalDelayBufferSize
  audioOut : Outport  VectorParamsAs1DForOutWhenUnconnected=off
  wires:
  delay_chain/1 -> PoolDelay/2
  audioIn/1 -> PoolDelay/1
  PoolDelay/1 -> audioOut/1

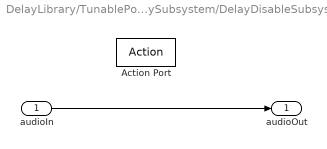
== system DelayLibrary/TunablePoolDelay/annDelaySubsystem/DelayDisableSubsystem ==
  audioIn : Inport
  Action Port : ActionPort
  audioOut : Outport  VectorParamsAs1DForOutWhenUnconnected=off
  wires:
  audioIn/1 -> audioOut/1

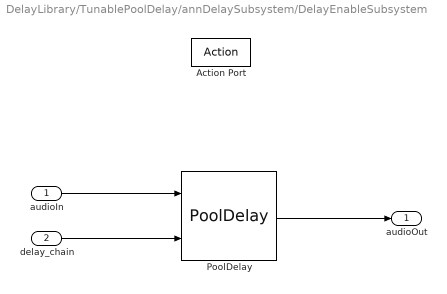
== system DelayLibrary/TunablePoolDelay/annDelaySubsystem/DelayEnableSubsystem ==
  audioIn : Inport
  delay_chain : Inport  Port=2
  Action Port : ActionPort
  PoolDelay : $bdroot/PoolDelay  variantSelect=L2 Memory  maxTotalDelay=maxTotalDelay  delayFrameLess=on  delayFrame=on  delayMultiFrame=on  frameSize=frameSize  numChannels=numChannels  totalDelayBufferSize=totalDelayBufferSize  totalFastDelayBufferSize=totalDelayBufferSize
  audioOut : Outport  VectorParamsAs1DForOutWhenUnconnected=off
  wires:
  PoolDelay/1 -> audioOut/1
  audioIn/1 -> PoolDelay/1
  delay_chain/1 -> PoolDelay/2

== matlab function DelayLibrary/TunablePoolDelay/DelayTranslation/translation ==
  data: Samples output; Amount input; sampleRate input; delayType parameter; maxTotalDelay parameter
  events: trigger input FUNCTION_CALL_EVENT
function Samples = fcn(Amount, sampleRate, delayType, maxTotalDelay)

if (delayType == 1) % delay in samples
    Samples = uint32(ceil(Amount.Value));
else % delay in milliseconds
    Samples = uint32(ceil(Amount.Value * 1e-3 * sampleRate));
end

% Check if Channel Delay is greater than max allowed pool delay
chanDelay = uint32(sum(Samples));
if (chanDelay > maxTotalDelay)
    TranslateError('Total delay is bigger than allotted delay');
end

== matlab function DelayLibrary/Shared Delay/shared delay init ==
  data: u input; delayChain input; inputMapping input; codeWorkMemory data_store_memory; delayBuffer data_store_memory; fastDmaBuffer data_store_memory
  events: trigger input FUNCTION_CALL_EVENT
function shared_delay_init(u, delayChain, inputMapping)
% Shared delay function provides multiple delay line tap outputs for each 
% input channel. 
% 
% Parameters:
%   u:               Input channels [frame size x number of inputs]
%   delayChain:      Delay in samples for each channel [1 x number of outputs]
%   inputMapping:    Zero-based input mapping for each filter [1 x number of outputs]
%
% Global parameters:
%   delayBuffer:     Delay line circular buffer containing all channel  
%                    delay state data
%   fastDmaBuffer:   Fast DMA buffer containing all channel outputs for
%                    next frame
%   codeWorkMemory:  Working memory set up during roommode reset/init CRL
%                    function call [1 x codeWorkMemorySize]

global delayBuffer;
global fastDmaBuffer;
global codeWorkMemory;

% Extract configuration information from input
[frameSize, numInputs]  = size(u);
numOutputs = numel(delayChain);

% Get the work memory and delay buffer sizes
workMemorySize = numel(codeWorkMemory);
delayBufferSize = numel(delayBuffer);
fastDmaBufferSize = numel(fastDmaBuffer);

% Set correct data types
frameSize = int32(frameSize);
numInputs = int32(numInputs);
numOutputs = int32(numOutputs);
delayChain = int32(delayChain);
inputMapping = int32(inputMapping);
workMemorySize = int32(workMemorySize);
delayBufferSize = int32(delayBufferSize);
fastDmaBufferSize = int32(fastDmaBufferSize);

% Initialization
y = shared_delay_mdma_init(u, delayBuffer, delayBufferSize, ...
                           fastDmaBuffer, fastDmaBufferSize, ...
                           delayChain, inputMapping, numInputs, ... 
                           numOutputs, frameSize, codeWorkMemory, ...
                           workMemorySize);

% NOTE: The CRL mechanism requires an output for the function call,
% and appears to be optimized out if that return value isn't used. 
% This is a dummy operation to make sure CRL ends up in generated code
codeWorkMemory(1) = y; 

end


% Shared delay CRL initialization function conceptual specification
function y = shared_delay_mdma_init(u, delayBuffer, delayBufferSize, ...
                                    fastDmaBuffer, fastDmaBufferSize, ...    
                                    delayChain, inputMapping, numInputs, ...
                                    numOutputs, frameSize, workMemory, ...
                                    workMemorySize) 
% If target == codegen, error out if no CRL found
coder.replace('-errorifnoreplacement');

% No init simulation code, but need to do something to ensure CRL does not
% get optimized out
y = single(workMemory(1) + 1);

end

== matlab function DelayLibrary/Shared Delay/shared delay process ==
  data: u input; delayChain input; inputMapping input; y output; codeWorkMemory data_store_memory; delayBuffer data_store_memory
function y = shared_delay_process(u, delayChain, inputMapping)
% Shared delay function provides multiple delay line tap outputs for each 
% input channel.   
%
% Parameters:
%   u:              Input channels [frame size x number of inputs]
%   delayChain:     Delay in samples for each channel [1 x number of outputs]
%   inputMapping:   Zero-based input mapping for each filter [1 x number of outputs]
%
% Global parameters:
%   delayBuffer:     Delay line circular buffer containing all channel  
%                    delay state data
%   codeWorkMemory:  Working memory set up during roommode reset/init CRL
%                    function call [1 x codeWorkMemorySize]

global delayBuffer;
global codeWorkMemory;

% Get the fast delay buffer sizes
delayBufferSize = numel(delayBuffer);

% Set correct data types
delayChain = int32(delayChain);
delayBufferSize = int32(delayBufferSize);

% Simulation
if(coder.target('MATLAB') || coder.target('Sfun'))
    
    y = SharedDelaySim(u, delayChain, inputMapping, delayBufferSize);        
    
% Code generation
else 
    
    y = shared_delay_mdma_process(u, delayChain, codeWorkMemory);

end

end


% Shared delay CRL step/process function conceptual specification
function y = shared_delay_mdma_process(u, delayChain, workMemory)
% If target == codegen, error out if no CRL found
coder.replace('-errorifnoreplacement');

[frameSize, ~] = size(u);
numOutputs = numel(delayChain);
y = single(zeros(frameSize, numOutputs));
end

== matlab function DelayLibrary/ControllablePoolDelay/MATLAB Function ==
  data: Amount input; Samples output; maxTotalDelay parameter; numChannels parameter
function Samples = fcn(Amount, maxTotalDelay, numChannels)

% Check if Channel Delay is greater than max allowed pool delay
if (Amount*numChannels > maxTotalDelay)
    Amount = uint32(floor(maxTotalDelay/numChannels));
end
Samples = Amount;

== matlab function DelayLibrary/PoolDelay/pool delay init ==
  data: u input; delayChain input; codeWorkMemory data_store_memory; variantSelect parameter; delayBuffer data_store_memory; fastDelayBuffer data_store_memory
  events: trigger input FUNCTION_CALL_EVENT
function pool_delay_init(u, delayChain, variantSelect)

% Pool delay function provides delay lines for N channels.  Core
% implementation provides delay of any positive integer value.  MDMA
% implementation provides integer value delays of a frame or greater. 
% 
% Parameters:
%   u:              Input channels [frame size x number of inputs]
%   delayChain:     Delay in samples for each channel [1 x delay per channel]
%   variantSelect:  Variant selection of implementation (scaler)
%
% Global parameters:
%   delayBuffer:    Delay line circular buffer containing all channel  
%                   delay state data
%   fastDelayBuffer: Fast delay line circular buffer containing all channel  
%                    delay state data
%   codeWorkMemory: Working memory set up during roommode reset/init CRL
%                   function call [1 x codeWorkMemorySize]

% Extract configuration information from inut
[frameSize, numChannels]  = size(u);

global delayBuffer;
global fastDelayBuffer;
global codeWorkMemory;

% Get the work memory and delay buffer sizes
workMemorySize = numel(codeWorkMemory);
delayBufferSize = numel(delayBuffer);
fastDelayBufferSize = numel(fastDelayBuffer);

% Set correct data types
frameSize = uint32(frameSize);
numChannels = uint32(numChannels);
delayChain = uint32(delayChain);
workMemorySize = uint32(workMemorySize);
delayBufferSize = uint32(delayBufferSize);
fastDelayBufferSize = uint32(fastDelayBufferSize);
    
% There are three implementation types:
% Type       Value     Description
% L1 Memory    1       Optimized CRL C code using L1 memory delay buffer and 
%                      core for movement of data in/out of delay buffer
% L2 Memory    2       Optimized CRL C code using L2 memory delay buffer and
%                      MDMA for movement of data in/out of delay buffer
% Generic      3       Generic implementation for other targets without CRL 
%
% NOTE: Generic implementation does not use codeWorkMemory, thus does not
% need any custom initialization.
if (variantSelect == 1)
    y = pool_delay_core_init(u, fastDelayBuffer, fastDelayBufferSize, ...
                             delayChain, numChannels, frameSize, ...
                             codeWorkMemory, workMemorySize);

                         
    % NOTE: The CRL mechanism requires an output for the function call,
    % and appears to be optimized out if that return value isn't used. 
    % This is a dummy operation to make sure CRL ends up in generated code
    codeWorkMemory(1) = y; 
elseif (variantSelect == 2)
    y = pool_delay_mdma_init(u, delayBuffer, delayBufferSize, ...
                             fastDelayBuffer, fastDelayBufferSize, ...
                             delayChain, numChannels, frameSize, ...
                             codeWorkMemory, workMemorySize);
    
    % NOTE: The CRL mechanism requires an output for the function call,
    % and appears to be optimized out if that return value isn't used. 
    % This is a dummy operation to make sure CRL ends up in generated code
    codeWorkMemory(1) = y; 
end

end


% Pool delay CRL core initialization function conceptual specification  
function y = pool_delay_core_init(u, fastDelayBuffer, fastDelayBufferSize, ... 
                                  delayChain, numChannels, frameSize, ...
                                  workMemory, workMemorySize)
% If target == codegen, error out if no CRL found
coder.replace('-errorifnoreplacement');

% No init simulation code, but need to do something to ensure CRL does not
% get optimized out
y = single(workMemory(1) + 1);

end


% Pool delay CRL MDMA initialization function conceptual specification
function y = pool_delay_mdma_init(u, delayBuffer, delayBufferSize, ...
                                  fastDelayBuffer, fastDelayBufferSize, ...
                                  delayChain, numChannels, frameSize, ...
                                  workMemory, workMemorySize) 
% If target == codegen, error out if no CRL found
coder.replace('-errorifnoreplacement');

% No init simulation code, but need to do something to ensure CRL does not
% get optimized out
y = single(workMemory(1) + 1);

end
